simulink model "ball_on_beam_final_template"  (R2022a)
settings: Solver=VariableStepAuto  StartTime=0.0  StopTime=20  RelTol=1e-3
undefined symbols (not defined in the file): A_e, B_e, C_e, k_fb, l_e
libraries: vrlib x4
settings Model: Creator=muellerb  LastModifiedBy=shard
settings DebuggingCC: UnconnectedInputMsg=warning  UnconnectedOutputMsg=warning  UnconnectedLineMsg=warning
settings RTWCC: DLArmComputeVersion=19.05

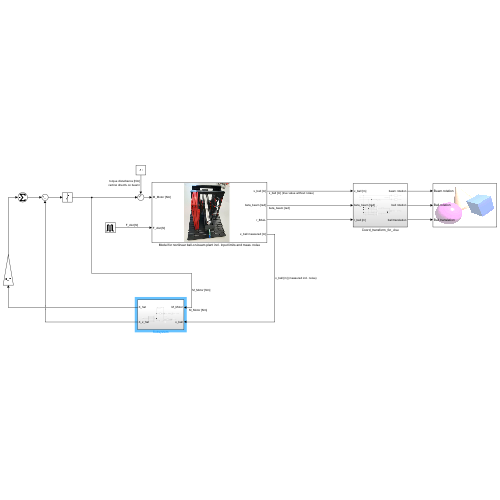
[thumbnail: Simulink's stored preview of the top-level diagram]
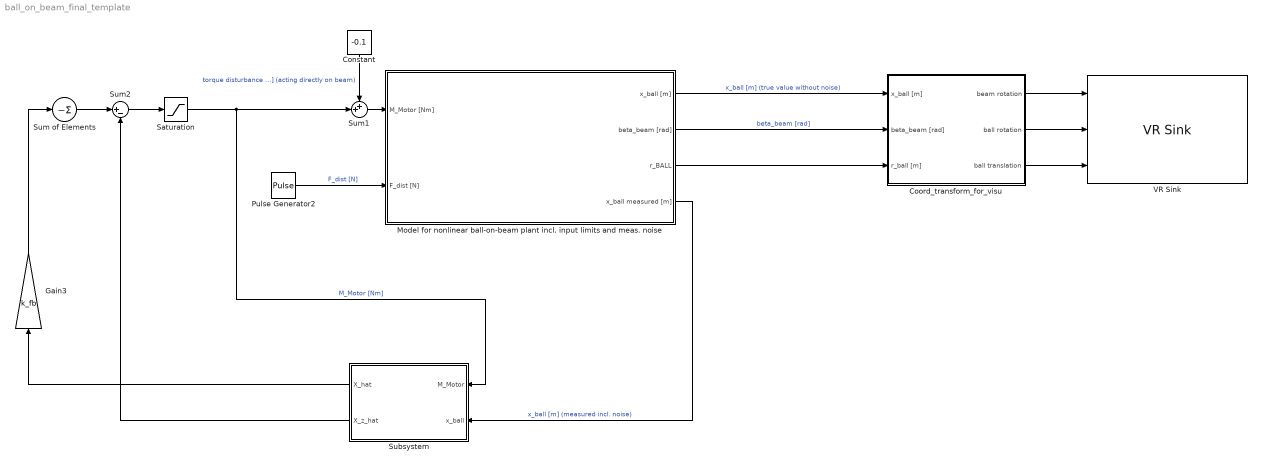
== system ball_on_beam_final_template ==
  Constant : Constant  Value=-0.1
  Coord_transform_for_visu : Subsystem
  Gain3 : Gain  Gain=k_fb
  Model for nonlinear ball-on-beam plant incl. input limits and meas. noise : Subsystem  mask(Nonlinear BALL_ON_BEAM model){r_BALL=0.0125, J_BALL=4.00e-06, m_BALL=0.064, G=9.81, J_BEAM=2.9e-3}
      mask prompts: r_BALL "Radius of the ball r_ball [m]"; J_BALL "Moment of inertia of the ball J_ball [kgm^2] (with respect to axis of symmetry)"; m_BALL "Mass of ball m_ball [kg]"; G "Gravity acceleration g [m/s^2]"; J_BEAM "Moment of inertia of the beam J_beam [kgm^2] (with respect to the axis of rotation)"
      mask help: Nonlinear model of ball-on-beam setup (without restrictions on input or state variables)
      mask Display: image('$imagefile'); % Use "Edit Image" on toolstrip to change.
  Pulse Generator2 : DiscretePulseGenerator  PulseType=Time based  Amplitude=2.5  Period=6  PulseWidth=0.06  PhaseDelay=3
  Saturation : Saturate  UpperLimit=0.6  LowerLimit=-0.6
  Subsystem : Subsystem
  Sum of Elements : Sum  Inputs=-
  Sum1 : Sum  Inputs=++|
  Sum2 : Sum  Inputs=|+-
  VR Sink : vrlib/VR Sink  InstantiateOnLoad=on  SampleTime=0.1  ViewEnable=on  RemoteChange=off  RemoteView=off  FieldsWritten=Beam.rotation.4.1.1.double#Ball.rotation.4.1.1.double#Ball.translation.3.1.1.double  WorldFileName=Ball_on_beam.wrl  AutoView=on  VideoDimensions=[]  AllowVariableSize=off
  wires:
  Pulse Generator2/1 -> Model for nonlinear ball-on-beam plant incl. input limits and meas. noise/2(F_dist [N])  "F_dist [N]"
  Model for nonlinear ball-on-beam plant incl. input limits and meas. noise/3(r_BALL) -> Coord_transform_for_visu/3(r_ball [m])
  Model for nonlinear ball-on-beam plant incl. input limits and meas. noise/1(x_ball [m]) -> Coord_transform_for_visu/1(x_ball [m])  "x_ball [m] (true value without noise)"
  Model for nonlinear ball-on-beam plant incl. input limits and meas. noise/2(beta_beam [rad]) -> Coord_transform_for_visu/2(beta_beam [rad])  "beta_beam [rad]"
  Saturation/1 -> Subsystem/1(M_Motor), Sum1/2  "M_Motor [Nm]"
  Coord_transform_for_visu/1(beam rotation) -> VR Sink/1
  Coord_transform_for_visu/2(ball rotation) -> VR Sink/2
  Coord_transform_for_visu/3(ball translation) -> VR Sink/3
  Subsystem/1(X_hat) -> Gain3/1
  Model for nonlinear ball-on-beam plant incl. input limits and meas. noise/4(x_ball measured [m]) -> Subsystem/2(x_ball)  "x_ball [m] (measured incl. noise)"
  Sum1/1 -> Model for nonlinear ball-on-beam plant incl. input limits and meas. noise/1(M_Motor [Nm])
  Constant/1 -> Sum1/1  "torque disturbance [Nm] (acting directly on beam)"
  Gain3/1 -> Sum of Elements/1
  Sum2/1 -> Saturation/1
  Subsystem/2(X_z_hat) -> Sum2/2
  Sum of Elements/1 -> Sum2/1

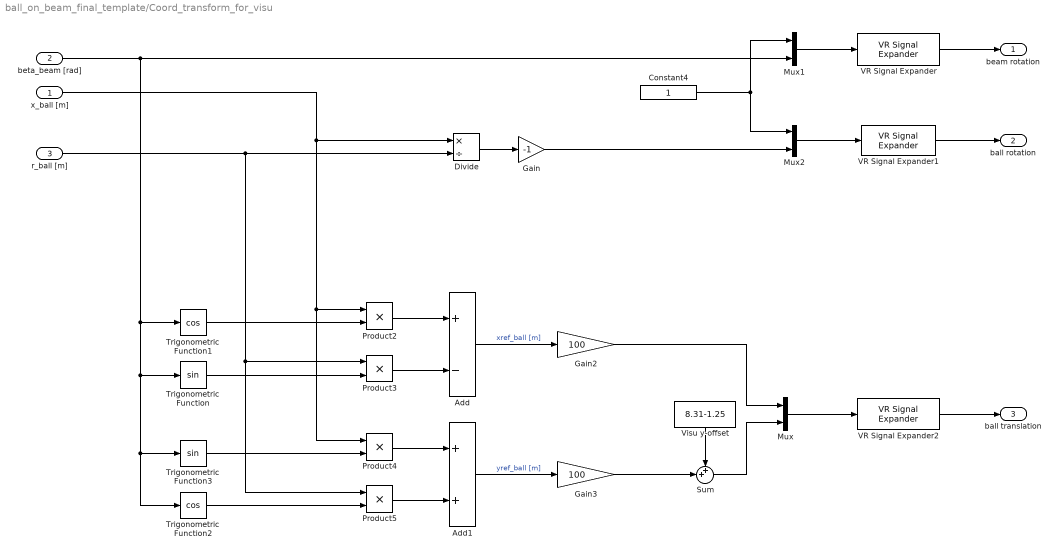
== system ball_on_beam_final_template/Coord_transform_for_visu ==
  x_ball [m] : Inport
  beta_beam [rad] : Inport  Port=2
  r_ball [m] : Inport  Port=3
  Add : Sum  Inputs=+-
  Add1 : Sum
  Constant4 : Constant
  Divide : Product  Inputs=*/
  Gain : Gain  Gain=-1
  Gain2 : Gain  Gain=100
  Gain3 : Gain  Gain=100
  Mux : Mux  Inputs=2
  Mux1 : Mux  Inputs=2
  Mux2 : Mux  Inputs=2
  Product{2..5} (4 alike) : Product
  Sum : Sum  Inputs=++|
  Trigonometric Function : Trigonometry
  Trigonometric Function1 : Trigonometry  Operator=cos
  Trigonometric Function2 : Trigonometry  Operator=cos
  Trigonometric Function3 : Trigonometry
  VR Signal Expander : vrlib/VR Signal Expander  outwidth=4  outidx=[3 4]
  VR Signal Expander1 : vrlib/VR Signal Expander  outwidth=4  outidx=[3 4]
  VR Signal Expander2 : vrlib/VR Signal Expander  outwidth=3  outidx=[1 2]
  Visu y-offset : Constant  Value=8.31-1.25
  beam rotation : Outport
  ball rotation : Outport  Port=2
  ball translation : Outport  Port=3
  wires:
  r_ball [m]/1 -> Divide/2, Product5/1, Product3/1
  Add/1 -> Gain2/1  "xref_ball [m]"
  x_ball [m]/1 -> Product4/1, Product2/1, Divide/1
  beta_beam [rad]/1 -> Mux1/2, Trigonometric Function1/1, Trigonometric Function2/1, Trigonometric Function3/1, Trigonometric Function/1
  Mux/1 -> VR Signal Expander2/1
  VR Signal Expander/1 -> beam rotation/1
  VR Signal Expander2/1 -> ball translation/1
  Trigonometric Function3/1 -> Product4/2
  Add1/1 -> Gain3/1  "yref_ball [m]"
  Gain/1 -> Mux2/2
  Mux2/1 -> VR Signal Expander1/1
  Constant4/1 -> Mux2/1, Mux1/1
  Trigonometric Function2/1 -> Product5/2
  Mux1/1 -> VR Signal Expander/1
  Divide/1 -> Gain/1
  Product4/1 -> Add1/1
  Visu y-offset/1 -> Sum/1
  Product5/1 -> Add1/2
  Gain2/1 -> Mux/1
  Product3/1 -> Add/2
  Trigonometric Function1/1 -> Product2/2
  Trigonometric Function/1 -> Product3/2
  Sum/1 -> Mux/2
  VR Signal Expander1/1 -> ball rotation/1
  Gain3/1 -> Sum/2
  Product2/1 -> Add/1

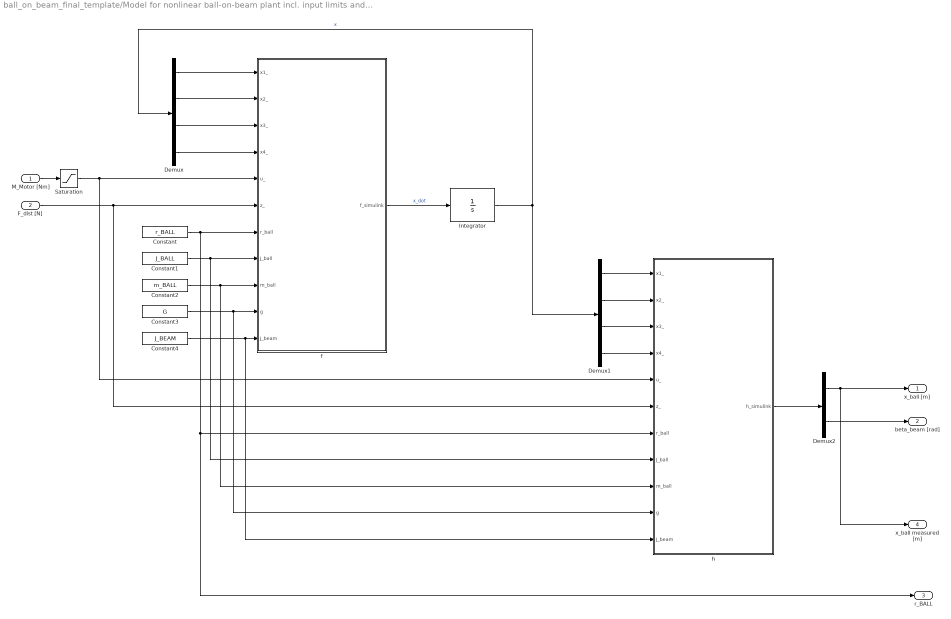
== system ball_on_beam_final_template/Model for nonlinear ball-on-beam plant incl. input limits and meas. noise ==
  M_Motor [Nm] : Inport
  F_dist [N] : Inport  Port=2
  Constant : Constant  Value=r_BALL
  Constant1 : Constant  Value=J_BALL
  Constant2 : Constant  Value=m_BALL
  Constant3 : Constant  Value=G
  Constant4 : Constant  Value=J_BEAM
  Demux : Demux
  Demux1 : Demux
  Demux2 : Demux  Outputs=2
  Integrator : Integrator
  Saturation : Saturate  UpperLimit=0.6  LowerLimit=-0.6
  f : MATLAB Function  TreatAsAtomicUnit=on
  h : MATLAB Function  TreatAsAtomicUnit=on
  x_ball [m] : Outport
  beta_beam [rad] : Outport  Port=2
  r_BALL : Outport  Port=3
  x_ball measured [m] : Outport  Port=4
  wires:
  Demux2/1 -> x_ball measured [m]/1, x_ball [m]/1
  M_Motor [Nm]/1 -> Saturation/1
  f/1(f_simulink) -> Integrator/1  "x_dot"
  h/1(h_simulink) -> Demux2/1
  Demux/3 -> f/3(x3_)
  Constant1/1 -> h/8(J_ball), f/8(J_ball)
  Demux/1 -> f/1(x1_)
  Integrator/1 -> Demux/1, Demux1/1  "x"
  F_dist [N]/1 -> h/6(z_), f/6(z_)
  Demux1/1 -> h/1(x1_)
  Constant4/1 -> h/11(J_beam), f/11(J_beam)
  Constant3/1 -> h/10(g), f/10(g)
  Constant/1 -> r_BALL/1, h/7(r_ball), f/7(r_ball)
  Demux2/2 -> beta_beam [rad]/1
  Constant2/1 -> h/9(m_ball), f/9(m_ball)
  Demux/2 -> f/2(x2_)
  Demux/4 -> f/4(x4_)
  Demux1/2 -> h/2(x2_)
  Demux1/3 -> h/3(x3_)
  Demux1/4 -> h/4(x4_)
  Saturation/1 -> h/5(u_), f/5(u_)

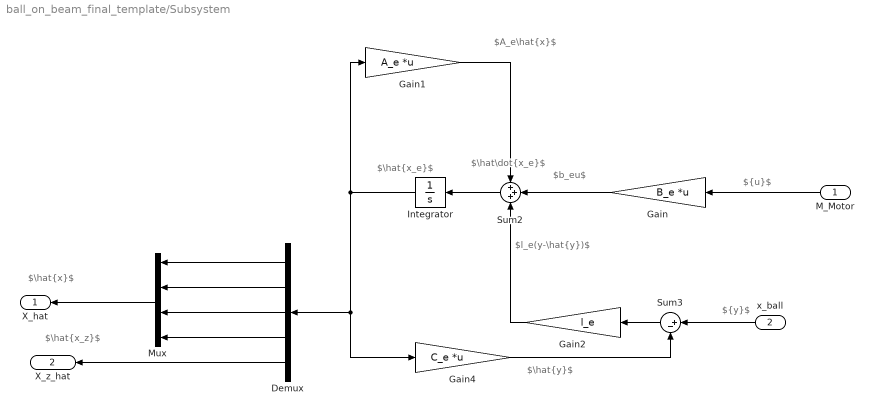
== system ball_on_beam_final_template/Subsystem ==
  note: $A_e\hat{x}$
  note: $b_eu$
  note: ${u}$
  note: $\hat{y}$
  note: ${y}$
  note: $l_e(y-\hat{y})$
  note: $\hat{x_e}$
  note: $\hat\dot{x_e}$
  note: $\hat{x}$
  note: $\hat{x_z}$
  M_Motor : Inport
  x_ball : Inport  Port=2
  Demux : Demux  Outputs=5
  Gain : Gain  Gain=B_e  Multiplication=Matrix(K*u)
  Gain1 : Gain  Gain=A_e  Multiplication=Matrix(K*u)
  Gain2 : Gain  Gain=l_e
  Gain4 : Gain  Gain=C_e  Multiplication=Matrix(K*u)
  Integrator : Integrator
  Mux : Mux
  Sum2 : Sum  Inputs=+++
  Sum3 : Sum  Inputs=|+-
  X_hat : Outport
  X_z_hat : Outport  Port=2
  wires:
  Integrator/1 -> Gain4/1, Demux/1, Gain1/1
  Gain4/1 -> Sum3/2
  Mux/1 -> X_hat/1
  x_ball/1 -> Sum3/1
  Sum3/1 -> Gain2/1
  Gain1/1 -> Sum2/1
  Gain/1 -> Sum2/2
  Sum2/1 -> Integrator/1
  Gain2/1 -> Sum2/3
  M_Motor/1 -> Gain/1
  Demux/1 -> Mux/1
  Demux/2 -> Mux/2
  Demux/3 -> Mux/3
  Demux/4 -> Mux/4
  Demux/5 -> X_z_hat/1

== matlab function ball_on_beam_final_template/Model for nonlinear ball-on-beam plant incl. input limits and meas. noise/f ==
  data: x1_ input; f_simulink output; x2_ input; x3_ input; x4_ input; u_ input; z_ input; r_ball input; J_ball input; m_ball input; g input; J_beam input
function f_simulink = f(x1_,x2_,x3_,x4_,u_,z_,r_ball,J_ball,m_ball,g,J_beam)
%#codegen

%    This function was generated by the Symbolic Math Toolbox version 8.7.
%    28-Nov-2023 16:51:32

t2 = cos(x3_);
t3 = sin(x3_);
t4 = m_ball.^2;
t5 = r_ball.^2;
t6 = x1_.^2;
t7 = x4_.^2;
t8 = m_ball.*t6;
t9 = J_beam+t8;
t10 = 1.0./t9;
f_simulink = [x2_;...
    (r_ball.*t10.*(J_ball.*u_+J_beam.*r_ball.*z_+m_ball.*t5.*u_+r_ball.*t8.*z_+r_ball.*t4.*t7.*x1_.^3+r_ball.^3.*t4.*t7.*x1_-J_beam.*g.*m_ball.*r_ball.*t3-J_ball.*g.*m_ball.*t2.*x1_+J_beam.*m_ball.*r_ball.*t7.*x1_+J_ball.*m_ball.*r_ball.*t7.*x1_-J_ball.*m_ball.*x1_.*x2_.*x4_.*2.0-g.*r_ball.*t3.*t4.*t6-g.*t2.*t4.*t5.*x1_-t4.*t5.*x1_.*x2_.*x4_.*2.0))./(J_ball+m_ball.*t5);x4_;t10.*(u_-g.*m_ball.*t2.*x1_+m_ball.*r_ball.*t7.*x1_-m_ball.*x1_.*x2_.*x4_.*2.0)];

== matlab function ball_on_beam_final_template/Model for nonlinear ball-on-beam plant incl. input limits and meas. noise/h ==
  data: x1_ input; h_simulink output; x2_ input; x3_ input; x4_ input; u_ input; z_ input; r_ball input; J_ball input; m_ball input; g input; J_beam input
function h_simulink = h(x1_,x2_,x3_,x4_,u_,z_,r_ball,J_ball,m_ball,g,J_beam)
%#codegen

%    This function was generated by the Symbolic Math Toolbox version 8.7.
%    28-Nov-2023 16:51:32

h_simulink = [x1_;...
    x3_];
